simulink model "matlab_model"  (R2017a)
settings: Solver=VariableStepAuto  StartTime=0.0  StopTime=10.0  RelTol=1e-3
libraries: mpclib x1
settings Model: Creator=gunge  LastModifiedBy=gunge

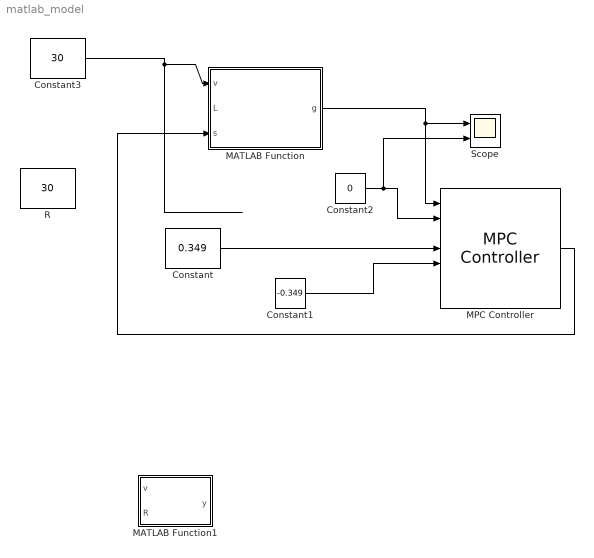
== system matlab_model ==
  Constant : Constant  Value=0.349
  Constant1 : Constant  Value=-0.349
  Constant2 : Constant  Value=0
  Constant3 : Constant  Value=30
  MATLAB Function : MATLAB Function  TreatAsAtomicUnit=on
  MATLAB Function1 : MATLAB Function  TreatAsAtomicUnit=on
  MPC Controller : mpclib/MPC Controller  SCDEnableBlockLinearizationSpecification=on  is_multiple=0  enable_value=0  return_u0=off  ref_from_ws=off  ref_signal_name=[]  ref_preview=off  md_from_ws=off  md_signal_name=[]  md_preview=off  from_project=off  project_file=MPCtask.mat  md_inport=on  mv_inport=off  cost_outport=off  return_sequence=off  return_qpstatus=off  return_state=off  state_inport=off  lims_inport=on  ywt_inport=off  is_designfromscratch=0  uwt_inport=off  duwt_inport=off  rhoeps_inport=off  uref_inport=off  n_ts=0.1  n_mv=1  n_md=1  n_ud=0  n_mo=1  n_uo=0  BlockDataType=double  SampleTimeInherited=off  switch_inport=off
  R : Constant  Value=30
  Scope : Scope  NumInputPorts=2
  wires:
  MATLAB Function/1(g) -> Scope/1, MPC Controller/1
  MPC Controller/1 -> MATLAB Function/3(s)
  Constant/1 -> MPC Controller/4
  Constant1/1 -> MPC Controller/5
  Constant2/1 -> Scope/2, MPC Controller/2
  Constant3/1 -> MATLAB Function/1(v)

== matlab function matlab_model/MATLAB Function1 ==
  data: v input; y output; R input
function y = fcn(v,R)


y = [0; 0; -v; 0]*1/R;

y = u;

== matlab function matlab_model/MATLAB Function ==
  data: v input; g output; L input; s input
function g = fcn(v,L, s)


% System parameters
m = 2023;       %kg
lf = 1.26;      %m
cf = 2.864e5;   %N/rad
J = 6286;       %kg.m2
lr = 1.90;      %m
cr = 1.948e5;   %N/rad

%% changable values    
%x0 = [ 0;0;0;y0];
%p_dis = 1/R; %1/R
v = v;         %m/sec
ls = L; % m
%%


a11 = -(cf+cr)/(m*v);
a12 = -1-(cf*lf-cr*lr)/(m*v^2);
a21 = -(cf*lf-cr*lr)/(J);
a22 = -(cf*lf^2 + cr*lr^2)/(J*v);
b1 = cf / (m*v);
b2 = cf*lf / J;
% Finite Horizon MPC as quadratic program
% State-Space Model of the System
Ac = [a11 a12 0 0;
      a21 a22 0 0; 
      0 1 0 0; 
      v ls v 0];
Bc = [b1; b2; 0; 0];
C =  [0 0 0 1];
D =  [0];
%dist = [0;0;-v;0]*p_dis;

%Bc = Bc-dist;

G = ss(Ac,Bc,C,D);

u1 = s;

X = [x1;x2;x3;x4];

X = Ac*X + Bc*u1;
Y = C*X + D*u1;

g = Y;
